simulink model "Exercitiul3"  (R2016a)
settings: Solver=VariableStepDiscrete  StartTime=0.0  StopTime=480  RelTol=1e-3
undefined symbols (not defined in the file): m, n
settings Model: Creator=Cristina  LastModifiedBy=Cristina

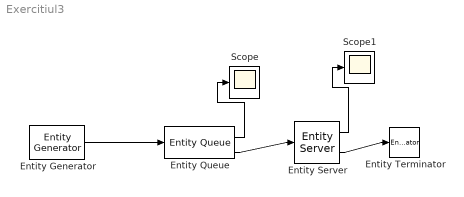
== system Exercitiul3 ==
  Entity Generator : EntityGenerator  OutputPortMessageModes=m  TimeSource=MATLAB action  IntergenerationTimeAction=dt = exprnd(0.2);  EntityType=Structured  EntityTypeName=Entity
  Entity Queue : EntityQueue  InputPortMessageModes=m  OutputPortMessageModes=n,m  AverageWait=on
      settings: OutputPortMap=o2,o5
  Entity Server : EntityServer  InputPortMessageModes=m  OutputPortMessageModes=n,m  ServiceTimeSource=MATLAB action  ServiceTimeAction=dt = 0.8 + 0.4 * rand;  Utilization=on
      settings: OutputPortMap=o5,o9
  Entity Terminator : EntityTerminator  InputPortMessageModes=m
  Scope : Scope
  Scope1 : Scope
  wires:
  Entity Queue/2 -> Entity Server/1
  Entity Generator/1 -> Entity Queue/1
  Entity Server/2 -> Entity Terminator/1
  Entity Queue/1 -> Scope/1
  Entity Server/1 -> Scope1/1
